simulink model "rotaryinvpend"  (R2019b)
settings: Solver=VariableStepAuto  StartTime=0.0  StopTime=10.0  RelTol=1e-3
values from neighbouring files (symbols this model uses):
  a = J+(m*r*r)    (= 0.028778125)    [ol_rip_linandnonlin_params.m]    (also in rotaryinvpend_params.m = 0.008078125)
  alpha_init = 0    [rotaryinvpend_params.m]
  b = m*L*r    (= 0.0045015625)    [ol_rip_linandnonlin_params.m]    (also in rotaryinvpend_params.m)
  c = (4/3)*m*L*L    (= 0.00467604166667)    [ol_rip_linandnonlin_params.m]    (also in rotaryinvpend_params.m)
  d = m*g*L    (= 0.205396875)    [ol_rip_linandnonlin_params.m]    (also in rotaryinvpend_params.m)
  e = Beq+(nm*ng*kt*kg*kg*km)/rm    (= 0.0844985569231)    [ol_rip_linandnonlin_params.m]    (also in rotaryinvpend_params.m)
  f = (nm*ng*kt*kg)/rm    (= 0.151313076923)    [ol_rip_linandnonlin_params.m]    (also in rotaryinvpend_params.m)
  k1 = -K(1)    [rotaryinvpend_params.m]
  k2 = -K(2)    [rotaryinvpend_params.m]
  k3 = -K(3)    [rotaryinvpend_params.m]
  k4 = -K(4)    [rotaryinvpend_params.m]
  theta_init = 0    [rotaryinvpend_params.m]
libraries: simulink x2
settings Model: Creator=SAI JOSHITHA  LastModifiedBy=SAI JOSHITHA

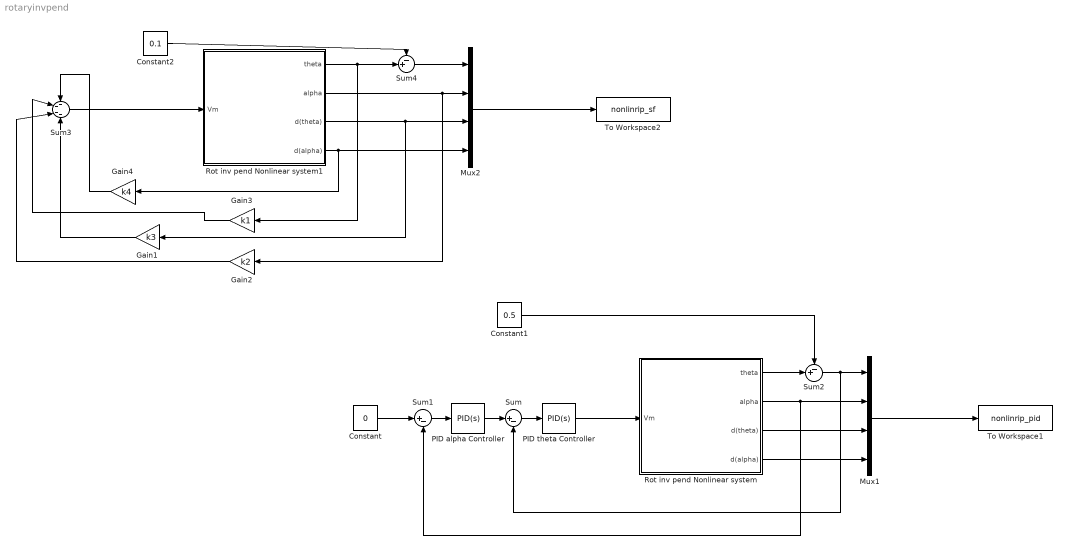
== system rotaryinvpend ==
  Constant : Constant  Value=0
  Constant1 : Constant  Value=0.5
  Constant2 : Constant  Value=0.1
  Gain1 : Gain  Gain=k3
  Gain2 : Gain  Gain=k2
  Gain3 : Gain  Gain=k1
  Gain4 : Gain  Gain=k4
  Mux1 : Mux
  Mux2 : Mux
  PID alpha Controller : simulink/Continuous/PID Controller  Controller=PID  Form=Parallel  TimeDomain=Continuous-time  SampleTime=-1  IntegratorMethod=Forward Euler  FilterMethod=Forward Euler  ControllerParametersSource=internal  P=104.8795  I=0.1049  D=0.4393  UseFilter=on  N=100  TunerSelectOption=Transfer Function Based (PID Tuner App)  InitialConditionSource=internal  InitialConditionForIntegrator=0  InitialConditionForFilter=0  DifferentiatorICPrevScaledInput=0  ExternalReset=none  TrackingMode=off  Kt=1  LimitOutput=off  UpperSaturationLimit=inf  LowerSaturationLimit=-inf  LinearizeAsGain=on  AntiWindupMode=none  Kb=1  POutMin=[]  POutMax=[]  IOutMin=[]  IOutMax=[]  DOutMin=[]  DOutMax=[]  NOutMin=[]  NOutMax=[]  SumOutMin=[]  SumOutMax=[]  SaturationOutMin=[]  SaturationOutMax=[]  PParamMin=[]  PParamMax=[]  IParamMin=[]  IParamMax=[]  DParamMin=[]  DParamMax=[]  NParamMin=[]  NParamMax=[]  KbParamMin=[]  KbParamMax=[]  KtParamMin=[]  KtParamMax=[]  KbOutMin=[]  KbOutMax=[]  KtOutMin=[]  KtOutMax=[]  IntegratorOutMin=[]  IntegratorOutMax=[]  FilterOutMin=[]  FilterOutMax=[]  SumI1OutMin=[]  SumI1OutMax=[]  SumI2OutMin=[]  SumI2OutMax=[]  SumI3OutMin=[]  SumI3OutMax=[]  SumI4OutMin=[]  SumI4OutMax=[]  SumDOutMin=[]  SumDOutMax=[]  DifferentiatorOutMin=[]  DifferentiatorOutMax=[]  FilterDiffOutCoefMin=[]  FilterDiffOutCoefMax=[]  ReciprocalOutMin=[]  ReciprocalOutMax=[]  SumDenOutMin=[]  SumDenOutMax=[]  SumNumOutMin=[]  SumNumOutMax=[]  DivideOutMin=[]  DivideOutMax=[]  IntegratorContinuousStateAttributes=''  IntegratorStateMustResolveToSignalObject=off  IntegratorRTWStateStorageClass=Auto  FilterContinuousStateAttributes=''  FilterStateMustResolveToSignalObject=off  FilterRTWStateStorageClass=Auto  ParallelPVariant=InternalParameters  IdealPVariant=Disabled  IVariant=InternalParameters  DVariant=InternalParameters  IntegratorVariant=Continuous  SatVariant=Disabled  AWVariant=Passthrough  PCopyVariant=Disabled  TRVariant=Disabled  FdbkBlocksVariant=Forward  IdealPFdbkVariant=Disabled  SatFdbkVariant=Disabled  DerivativeFilterVariant=ContFilter  NVariant=InternalParameters  NCopyVariant=Disabled  FilterICVariant=InternalICsFilter  IntegratorICVariant=InternalICs  ExternalResetVariant=Disabled  TRSumVariant=Passthrough  SumFdbkVariant=Disabled  SumVariant=Sum_PID
  PID theta Controller : simulink/Continuous/PID Controller  Controller=PID  Form=Parallel  TimeDomain=Continuous-time  SampleTime=-1  IntegratorMethod=Forward Euler  FilterMethod=Forward Euler  ControllerParametersSource=internal  P=264.1355  I=0.26413  D=3.7141  UseFilter=on  N=100  TunerSelectOption=Transfer Function Based (PID Tuner App)  InitialConditionSource=internal  InitialConditionForIntegrator=0  InitialConditionForFilter=0  DifferentiatorICPrevScaledInput=0  ExternalReset=none  TrackingMode=off  Kt=1  LimitOutput=off  UpperSaturationLimit=inf  LowerSaturationLimit=-inf  LinearizeAsGain=on  AntiWindupMode=none  Kb=1  POutMin=[]  POutMax=[]  IOutMin=[]  IOutMax=[]  DOutMin=[]  DOutMax=[]  NOutMin=[]  NOutMax=[]  SumOutMin=[]  SumOutMax=[]  SaturationOutMin=[]  SaturationOutMax=[]  PParamMin=[]  PParamMax=[]  IParamMin=[]  IParamMax=[]  DParamMin=[]  DParamMax=[]  NParamMin=[]  NParamMax=[]  KbParamMin=[]  KbParamMax=[]  KtParamMin=[]  KtParamMax=[]  KbOutMin=[]  KbOutMax=[]  KtOutMin=[]  KtOutMax=[]  IntegratorOutMin=[]  IntegratorOutMax=[]  FilterOutMin=[]  FilterOutMax=[]  SumI1OutMin=[]  SumI1OutMax=[]  SumI2OutMin=[]  SumI2OutMax=[]  SumI3OutMin=[]  SumI3OutMax=[]  SumI4OutMin=[]  SumI4OutMax=[]  SumDOutMin=[]  SumDOutMax=[]  DifferentiatorOutMin=[]  DifferentiatorOutMax=[]  FilterDiffOutCoefMin=[]  FilterDiffOutCoefMax=[]  ReciprocalOutMin=[]  ReciprocalOutMax=[]  SumDenOutMin=[]  SumDenOutMax=[]  SumNumOutMin=[]  SumNumOutMax=[]  DivideOutMin=[]  DivideOutMax=[]  IntegratorContinuousStateAttributes=''  IntegratorStateMustResolveToSignalObject=off  IntegratorRTWStateStorageClass=Auto  FilterContinuousStateAttributes=''  FilterStateMustResolveToSignalObject=off  FilterRTWStateStorageClass=Auto  ParallelPVariant=InternalParameters  IdealPVariant=Disabled  IVariant=InternalParameters  DVariant=InternalParameters  IntegratorVariant=Continuous  SatVariant=Disabled  AWVariant=Passthrough  PCopyVariant=Disabled  TRVariant=Disabled  FdbkBlocksVariant=Forward  IdealPFdbkVariant=Disabled  SatFdbkVariant=Disabled  DerivativeFilterVariant=ContFilter  NVariant=InternalParameters  NCopyVariant=Disabled  FilterICVariant=InternalICsFilter  IntegratorICVariant=InternalICs  ExternalResetVariant=Disabled  TRSumVariant=Passthrough  SumFdbkVariant=Disabled  SumVariant=Sum_PID
  Rot inv pend Nonlinear system : Subsystem
  Rot inv pend Nonlinear system1 : Subsystem
  Sum : Sum  Inputs=|+-
  Sum1 : Sum  Inputs=|+-
  Sum2 : Sum  Inputs=-+|
  Sum3 : Sum  Inputs=----
  Sum4 : Sum  Inputs=-+|
  To Workspace1 : ToWorkspace  VariableName=nonlinrip_pid  SaveFormat=Timeseries  SampleTime=-1
  To Workspace2 : ToWorkspace  VariableName=nonlinrip_sf  SaveFormat=Timeseries  SampleTime=-1
  wires:
  Rot inv pend Nonlinear system/4(d(alpha)) -> Mux1/4
  Rot inv pend Nonlinear system/1(theta) -> Sum2/2
  Rot inv pend Nonlinear system/3(d(theta)) -> Mux1/3
  Mux1/1 -> To Workspace1/1
  PID theta Controller/1 -> Rot inv pend Nonlinear system/1(Vm)
  Sum/1 -> PID theta Controller/1
  PID alpha Controller/1 -> Sum/1
  Sum1/1 -> PID alpha Controller/1
  Constant/1 -> Sum1/1
  Constant1/1 -> Sum2/1
  Rot inv pend Nonlinear system1/2(alpha) -> Gain2/1, Mux2/2
  Rot inv pend Nonlinear system1/1(theta) -> Sum4/2, Gain3/1
  Rot inv pend Nonlinear system1/3(d(theta)) -> Gain1/1, Mux2/3
  Rot inv pend Nonlinear system1/4(d(alpha)) -> Gain4/1, Mux2/4
  Mux2/1 -> To Workspace2/1
  Gain1/1 -> Sum3/4
  Gain2/1 -> Sum3/3
  Gain3/1 -> Sum3/2
  Gain4/1 -> Sum3/1
  Sum3/1 -> Rot inv pend Nonlinear system1/1(Vm)
  Sum4/1 -> Mux2/1
  Constant2/1 -> Sum4/1
  Sum2/1 -> Sum/2, Mux1/1
  Rot inv pend Nonlinear system/2(alpha) -> Mux1/2, Sum1/2

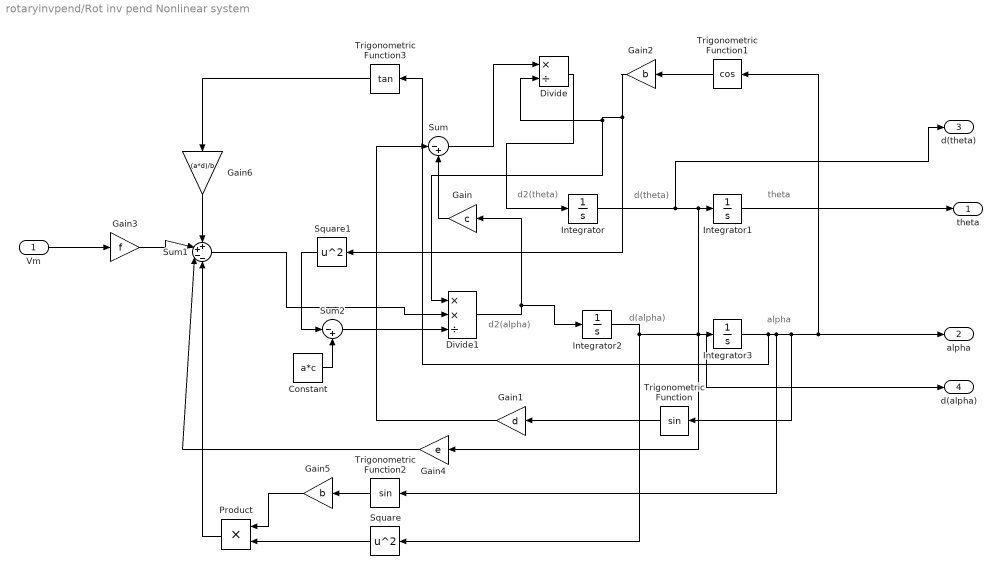
== system rotaryinvpend/Rot inv pend Nonlinear system ==
  note: d2(alpha)
  note: d(alpha)
  note: alpha
  note: d2(theta)
  note: d(theta)
  note: theta
  Vm : Inport
  Constant : Constant  Value=a*c
  Divide : Product  Inputs=*/
  Divide1 : Product  Inputs=**/
  Gain : Gain  Gain=c
  Gain1 : Gain  Gain=d
  Gain2 : Gain  Gain=b
  Gain3 : Gain  Gain=f
  Gain4 : Gain  Gain=e
  Gain5 : Gain  Gain=b
  Gain6 : Gain  Gain=(a*d)/b
  Integrator : Integrator
  Integrator1 : Integrator  InitialCondition=theta_init
  Integrator2 : Integrator
  Integrator3 : Integrator  InitialCondition=alpha_init
  Product : Product
  Square : Math  Operator=square  SignedPower=off  SaturateOnIntegerOverflow=on
  Square1 : Math  Operator=square  SignedPower=off  SaturateOnIntegerOverflow=on
  Sum : Sum  Inputs=|-+
  Sum1 : Sum  Inputs=++--
  Sum2 : Sum  Inputs=|-+
  Trigonometric Function : Trigonometry
  Trigonometric Function1 : Trigonometry  Operator=cos
  Trigonometric Function2 : Trigonometry
  Trigonometric Function3 : Trigonometry  Operator=tan
  theta : Outport
  alpha : Outport  Port=2
  d(theta) : Outport  Port=3
  d(alpha) : Outport  Port=4
  wires:
  Vm/1 -> Gain3/1
  Integrator2/1 -> Square/1, Integrator3/1, d(alpha)/1
  Integrator/1 -> d(theta)/1, Gain4/1, Integrator1/1
  Integrator3/1 -> Trigonometric Function3/1, Trigonometric Function2/1, Trigonometric Function1/1, alpha/1, Trigonometric Function/1
  Integrator1/1 -> theta/1
  Gain/1 -> Sum/2
  Trigonometric Function/1 -> Gain1/1
  Gain1/1 -> Sum/1
  Trigonometric Function1/1 -> Gain2/1
  Sum/1 -> Divide/1
  Gain2/1 -> Square1/1, Divide1/1, Divide/2
  Divide/1 -> Integrator/1
  Gain3/1 -> Sum1/2
  Gain4/1 -> Sum1/3
  Trigonometric Function2/1 -> Gain5/1
  Gain5/1 -> Product/1
  Square/1 -> Product/2
  Product/1 -> Sum1/4
  Trigonometric Function3/1 -> Gain6/1
  Gain6/1 -> Sum1/1
  Divide1/1 -> Gain/1, Integrator2/1
  Square1/1 -> Sum2/1
  Sum1/1 -> Divide1/2
  Sum2/1 -> Divide1/3
  Constant/1 -> Sum2/2

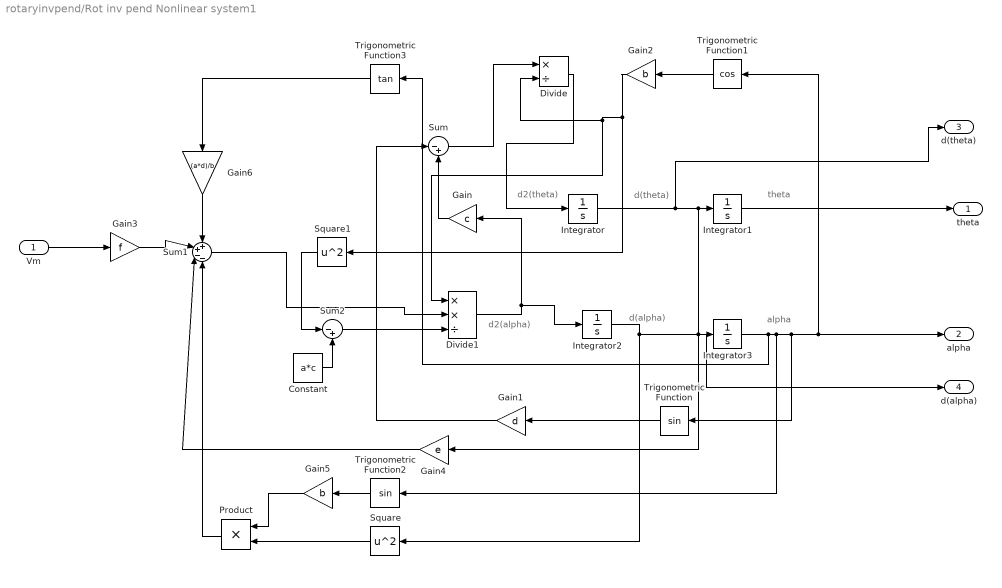
== system rotaryinvpend/Rot inv pend Nonlinear system1 ==
  note: d2(alpha)
  note: d(alpha)
  note: alpha
  note: d2(theta)
  note: d(theta)
  note: theta
  Vm : Inport
  Constant : Constant  Value=a*c
  Divide : Product  Inputs=*/
  Divide1 : Product  Inputs=**/
  Gain : Gain  Gain=c
  Gain1 : Gain  Gain=d
  Gain2 : Gain  Gain=b
  Gain3 : Gain  Gain=f
  Gain4 : Gain  Gain=e
  Gain5 : Gain  Gain=b
  Gain6 : Gain  Gain=(a*d)/b
  Integrator : Integrator
  Integrator1 : Integrator  InitialCondition=theta_init
  Integrator2 : Integrator
  Integrator3 : Integrator  InitialCondition=alpha_init
  Product : Product
  Square : Math  Operator=square  SignedPower=off  SaturateOnIntegerOverflow=on
  Square1 : Math  Operator=square  SignedPower=off  SaturateOnIntegerOverflow=on
  Sum : Sum  Inputs=|-+
  Sum1 : Sum  Inputs=++--
  Sum2 : Sum  Inputs=|-+
  Trigonometric Function : Trigonometry
  Trigonometric Function1 : Trigonometry  Operator=cos
  Trigonometric Function2 : Trigonometry
  Trigonometric Function3 : Trigonometry  Operator=tan
  theta : Outport
  alpha : Outport  Port=2
  d(theta) : Outport  Port=3
  d(alpha) : Outport  Port=4
  wires:
  Vm/1 -> Gain3/1
  Integrator2/1 -> Square/1, Integrator3/1, d(alpha)/1
  Integrator/1 -> d(theta)/1, Gain4/1, Integrator1/1
  Integrator3/1 -> Trigonometric Function3/1, Trigonometric Function2/1, Trigonometric Function1/1, alpha/1, Trigonometric Function/1
  Integrator1/1 -> theta/1
  Gain/1 -> Sum/2
  Trigonometric Function/1 -> Gain1/1
  Gain1/1 -> Sum/1
  Trigonometric Function1/1 -> Gain2/1
  Sum/1 -> Divide/1
  Gain2/1 -> Square1/1, Divide1/1, Divide/2
  Divide/1 -> Integrator/1
  Gain3/1 -> Sum1/2
  Gain4/1 -> Sum1/3
  Trigonometric Function2/1 -> Gain5/1
  Gain5/1 -> Product/1
  Square/1 -> Product/2
  Product/1 -> Sum1/4
  Trigonometric Function3/1 -> Gain6/1
  Gain6/1 -> Sum1/1
  Divide1/1 -> Gain/1, Integrator2/1
  Square1/1 -> Sum2/1
  Sum1/1 -> Divide1/2
  Sum2/1 -> Divide1/3
  Constant/1 -> Sum2/2
